simulink model "dbuildv3p2"  (R2024b)
settings: Solver=FixedStepAuto  StartTime=0.0  StopTime=inf  FixedStep=0.001  RelTol=1e-3
model workspace (MAT data in the model file):
  A_busbar = 0.0018
  A_pack = 0.711626248
  C = 400
  C_nominal = 3
  GR = 13.75
  I_max = 157.708978328
  Izz = 76.97
  M = 251.54
  P = 5
  P_DD = 1
  REGEN_GAIN = 0
  R_e = 0.197
  S = 138
  SW_TV_GAIN = 0.0250298750679
  SoC_initial = 1
  TC_CUT = 500
  T_amb = 296.15
  Tmax = 21
  W = 1.53
  W_max = 34
  a = 0.7497
  brakebias = 0.5
  busbar_CC_area = 1.8e-05
  busbar_Cp = 237
  busbar_length = 0.1
  busbar_mass = 0.016128
  busbar_resistivity = 1.68e-08
  busbar_thermalcontact_resistance = 1
  c_factor = 0.244
  cell_Cp = 1000
  cell_mass = 0.046
  deg_to_rad = 0.0174533
  g = 9.81
  h = 0.253
  h_busbar = 5
  h_pack = 5
  kappa_thresh = 0.09
  l = 1.53
  mpersec_to_kph = 3.6
  rackdisp_to_steerangle = 1.29615626969
  rad_to_deg = 57.2958
  rpm_to_radpers = 0.10472
  t = 1.2
  trigger_pressure = 4.65396
undefined symbols (not defined in the file): TC_switch, TV_switch
libraries: eeGeneralControl x2, Solver_SF x1, sl3dlib x1, simulink x1
(part 1 of 2)
settings Model: Creator=account  LastModifiedBy=kara.28

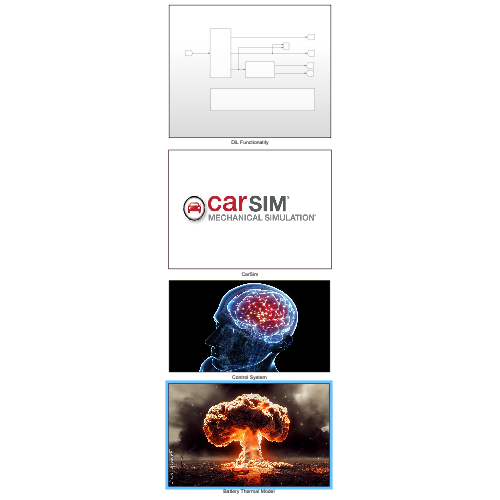
[thumbnail: Simulink's stored preview of the top-level diagram]
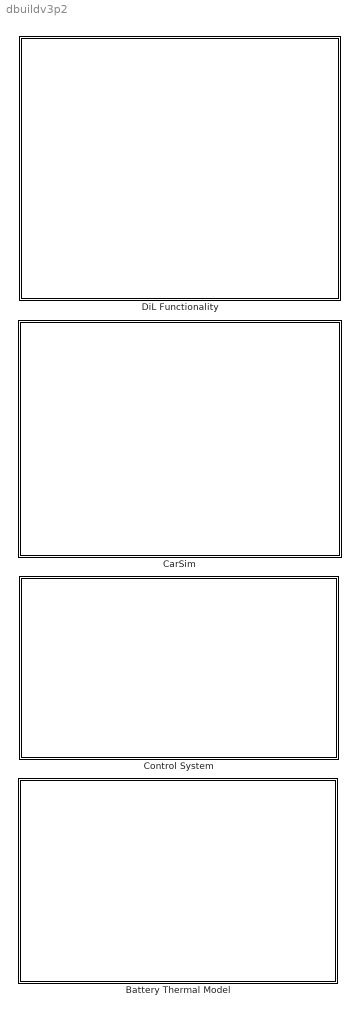
== system dbuildv3p2 ==
  Battery Thermal Model : Subsystem
      mask Display: image('battery.jpg');
  CarSim : Subsystem
      mask Display: image('carsimlogo.jpg');
  Control System : Subsystem
      mask Display: image('controller.jpg');
  DiL Functionality : Subsystem

== system dbuildv3p2/Battery Thermal Model ==
  Air Temp : Subsystem
  Battery Cells : Subsystem
  Bus Bars : Subsystem

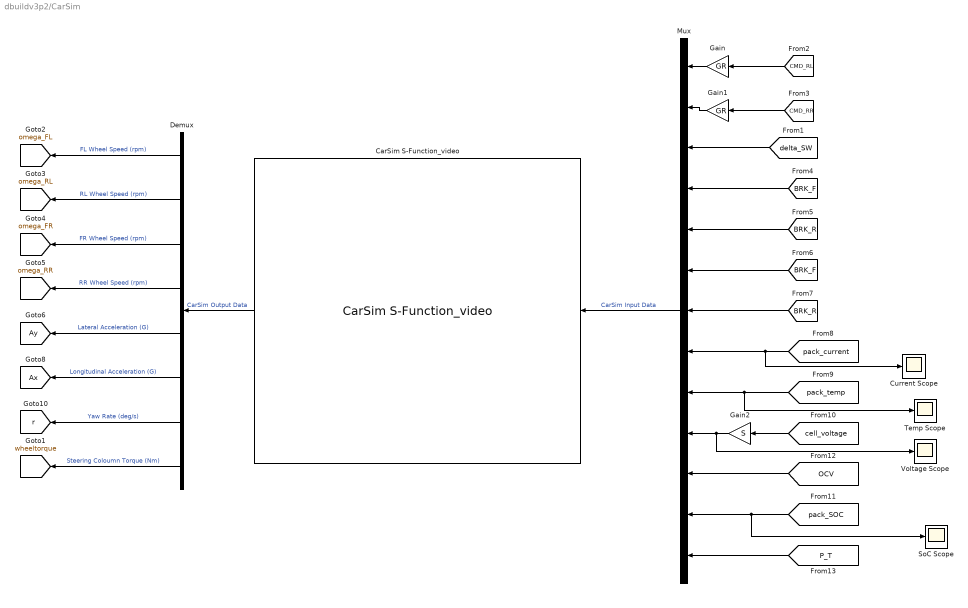
== system dbuildv3p2/CarSim ==
  CarSim S-Function_video : Solver_SF/CarSim S-Function_video  Priority=1  SIMFILE=simfile.sim
      settings: SourceProductName=CarSim S-Function
  Current Scope : Scope
  Demux : Demux  Outputs=8
  Gain : Gain  Gain=GR
  Gain1 : Gain  Gain=GR
  Gain2 : Gain  Gain=S
  Mux : Mux  Inputs=13
  SoC Scope : Scope
  Temp Scope : Scope
  Voltage Scope : Scope
  tag scope: Ax=global, Ay=global, omega_FL=global, omega_FR=global, omega_RL=global, omega_RR=global, r=global, wheeltorque=global
  wires:
  CarSim S-Function_video/1 -> Demux/1  "CarSim Output Data"
  [BRK_F] -> Mux/6
  Gain/1 -> Mux/1
  [pack_current] -> Current Scope/1, Mux/8
  Mux/1 -> CarSim S-Function_video/1  "CarSim Input Data"
  [BRK_R] -> Mux/7
  Gain1/1 -> Mux/2
  [BRK_R] -> Mux/5
  [BRK_F] -> Mux/4
  [delta_SW] -> Mux/3
  Demux/1 -> [omega_FL]  "FL Wheel Speed (rpm)"
  Demux/2 -> [omega_RL]  "RL Wheel Speed (rpm)"
  Demux/3 -> [omega_FR]  "FR Wheel Speed (rpm)"
  Demux/4 -> [omega_RR]  "RR Wheel Speed (rpm)"
  Demux/5 -> [Ay]  "Lateral Acceleration (G)"
  Demux/6 -> [Ax]  "Longitudinal Acceleration (G)"
  Demux/7 -> [r]  "Yaw Rate (deg/s)"
  Demux/8 -> [wheeltorque]  "Steering Coloumn Torque (Nm)"
  [pack_SOC] -> SoC Scope/1, Mux/12
  [OCV] -> Mux/11
  [cell_voltage] -> Gain2/1
  [pack_temp] -> Temp Scope/1, Mux/9
  Gain2/1 -> Voltage Scope/1, Mux/10
  [CMD_RL] -> Gain/1
  [CMD_RR] -> Gain1/1
  [P_T] -> Mux/13

== system dbuildv3p2/Control System ==
  Driver Assists : Subsystem
      settings: PortSchema="{\"entries\":[{\"content\":{\"sides\":[{\"content\":{\"connectorIds\":[\"In1\",\"In2\"]},\"type\":\"ConnectorPlacement.EquallySpacedRectSide\",\"uuid\":\"c30f5bbb-5f7b-4b8f-a220-579b9cc0865f\"},{\"content\":{\"connectorIds\":[\"Out1\",\"Out2\"],\"side\":\"RIGHT\"},\"type\":\"ConnectorPlacement.EquallySpacedRectSide\",\"uuid\":\"8399a92e-19c3-49c4-801c-f7e7f76799cf\"},{\"content\":{\"connectorIds\":[\"In3\",\"In4\",\"In5\",\"In6\",\"In7\",\"In8\",\"In9\"],\"side\":\"TOP\"},\"type\":\"ConnectorPlacement.EquallySpacedRectSide\",\"uuid\":\"19d8375b-8353-4f23-adee-fcd0b0fbd4ef\"}]},\"type\":\"ConnectorPlacement.EquallySpacedConnector\",\"uuid\":\"53834b5a-6686-42bc-a078-9cae71bfd001\"}],\"packageUris\":[\"http://schema.mathworks.com/mf0/Connector/R2020b\"],\"version\":\"1.0\"}"
  Dynamic Derate Dial Position : Constant  Value=3
  Energy Management System : Subsystem
      settings: PortSchema="{\"entries\":[{\"content\":{\"sides\":[{\"content\":{\"connectorIds\":[\"In1\",\"In2\"]},\"type\":\"ConnectorPlacement.EquallySpacedRectSide\",\"uuid\":\"89c92abe-ca77-4c48-ba79-1fd8447b36ee\"},{\"content\":{\"connectorIds\":[\"Out1\",\"Out2\"],\"side\":\"RIGHT\"},\"type\":\"ConnectorPlacement.EquallySpacedRectSide\",\"uuid\":\"4a58accb-bbe3-490f-b1ea-5257f75ab2ba\"},{\"content\":{\"connectorIds\":[\"In3\",\"In4\",\"In5\"],\"side\":\"TOP\"},\"type\":\"ConnectorPlacement.EquallySpacedRectSide\",\"uuid\":\"b5e96e52-1098-4ccd-9740-b2b10d8cf6b3\"}]},\"type\":\"ConnectorPlacement.EquallySpacedConnector\",\"uuid\":\"06c6d35a-fc7b-4382-b862-8bbe65743431\"}],\"packageUris\":[\"http://schema.mathworks.com/mf0/Connector/R2020b\"],\"version\":\"1.0\"}"
  tag scope: CMD_RL=global, CMD_RR=global
  wires:
  Energy Management System/1(CMD_R) -> Driver Assists/1(CMD_R)
  Energy Management System/2(Tmax) -> Driver Assists/2(Tmax)
  Driver Assists/1(CMD_RL) -> [CMD_RL]
  Driver Assists/2(CMD_RR) -> [CMD_RR]
  [pack_temp] -> Energy Management System/1(T_BAT_MAX)  "Battery Temp (C)"
  Dynamic Derate Dial Position/1 -> Energy Management System/2(P_DD)  "Derate Dial Position (-)"
  [omega_RR] -> Driver Assists/6(omega_RR), Energy Management System/5(omega_RR)  "RR Wheel Speed (rpm)"
  [omega_FR] -> Driver Assists/4(omega_FR)  "FR Wheel Speed (rpm)"
  [omega_RL] -> Driver Assists/5(omega_RL), Energy Management System/3(omega_RL)  "RL Wheel Speed (rpm)"
  [omega_FL] -> Driver Assists/3(omega_FL)  "FL Wheel Speed (rpm)"
  [P_T] -> Driver Assists/7(P_T)  "Throttle Position (-)"
  [Ay] -> Driver Assists/8(Ax)  "Lateral Acceleration (G)"
  [BRK_F] -> Driver Assists/9(BRK_F), Energy Management System/4(BRK_F)  "Front Brake Pressure (MPa)"

== system dbuildv3p2/DiL Functionality ==
  Brake system : Subsystem
  Driver inputs : Subsystem
  Real Time Sync : Subsystem
  Scope : Scope  NumInputPorts=2
  tag scope: BRK_F=global, BRK_R=global, P_T=global, delta_SW=global
  wires:
  Driver inputs/2(Throttle %) -> Scope/1, [P_T]  "Throttle (-)"
  Driver inputs/1(Steering) -> [delta_SW]  "Steering Angle (deg)"
  [wheeltorque] -> Driver inputs/1(Wheel torque)
  Brake system/1(Front brake pressure) -> [BRK_F]  "Front Brake Pressure (MPa)"
  Brake system/2(Rear brake pressure) -> [BRK_R]  "Front Brake Pressure (MPa)"
  Driver inputs/3(Brake %) -> Brake system/1(brake %), Scope/2  "Brake (-)"

== system dbuildv3p2/Battery Thermal Model/Air Temp ==
  Constant : Constant  Value=0.25
  Constant1 : Constant  Value=1005
  Constant2 : Constant  Value=T_amb
  Divide : Product  Inputs=*/
  Integrator : Integrator
  Product : Product
  Sum : Sum  Inputs=|++
  tag scope: airtemp=global
  wires:
  [pack_heatloss] -> Divide/1
  Product/1 -> Divide/2
  Constant/1 -> Product/2
  Constant1/1 -> Product/1
  Divide/1 -> Integrator/1
  Integrator/1 -> Sum/1
  Constant2/1 -> Sum/2
  Sum/1 -> [airtemp]

== system dbuildv3p2/Battery Thermal Model/Battery Cells ==
  Battery Heat : Subsystem
      settings: PortSchema="{\"entries\":[{\"content\":{\"sides\":[{\"content\":{\"connectorIds\":[\"In1\",\"Out1\",\"In2\"]},\"type\":\"ConnectorPlacement.EquallySpacedRectSide\",\"uuid\":\"0f7c0562-63f7-413a-9c65-7d5d0f23ac53\"},{\"content\":{\"side\":\"RIGHT\"},\"type\":\"ConnectorPlacement.EquallySpacedRectSide\",\"uuid\":\"6856fc4a-e601-47fb-aafe-3183d6398fa2\"},{\"content\":{\"side\":\"TOP\"},\"type\":\"ConnectorPlacement.EquallySpacedRectSide\",\"uuid\":\"93500152-ab0c-4e86-a765-8796b82b9cd6\"}]},\"type\":\"ConnectorPlacement.EquallySpacedConnector\",\"uuid\":\"8bef09a8-0835-4033-ba4e-3f5f6277d0ac\"}],\"packageUris\":[\"http://schema.mathworks.com/mf0/Connector/R2020b\"],\"version\":\"1.0\"}"
  Battery Heat Generation : Subsystem
  Heat Loss : Subsystem
      settings: PortSchema="{\"entries\":[{\"content\":{\"sides\":[{\"content\":{},\"type\":\"ConnectorPlacement.EquallySpacedRectSide\",\"uuid\":\"cd11f8f0-ebc0-4dda-8c98-00f5919de41a\"},{\"content\":{\"connectorIds\":[\"In1\",\"Out1\"],\"side\":\"RIGHT\"},\"type\":\"ConnectorPlacement.EquallySpacedRectSide\",\"uuid\":\"2a68a9a1-bd97-4a17-8a8b-1aa98e9bd9a8\"},{\"content\":{\"side\":\"TOP\"},\"type\":\"ConnectorPlacement.EquallySpacedRectSide\",\"uuid\":\"debcc510-941b-4448-a371-f67c84c59f32\"}]},\"type\":\"ConnectorPlacement.EquallySpacedConnector\",\"uuid\":\"91559e46-754b-48b4-ac3e-ab135f9add0a\"}],\"packageUris\":[\"http://schema.mathworks.com/mf0/Connector/R2020b\"],\"version\":\"1.0\"}"
  wires:
  Battery Heat/1(Pack Temp (K)) -> Heat Loss/1(Pack Temp (K))
  Battery Heat Generation/1(Battery Heat Generation Rate) -> Battery Heat/1(Battery Heat Generation)
  Heat Loss/1(Pack Heat Loss Rate) -> Battery Heat/2(Battery Heat Loss)

== system dbuildv3p2/Battery Thermal Model/Bus Bars ==
  Ambient Heat Loss : Subsystem
      settings: PortSchema="{\"entries\":[{\"content\":{\"sides\":[{\"content\":{},\"type\":\"ConnectorPlacement.EquallySpacedRectSide\",\"uuid\":\"cd11f8f0-ebc0-4dda-8c98-00f5919de41a\"},{\"content\":{\"connectorIds\":[\"In1\",\"Out1\"],\"side\":\"RIGHT\"},\"type\":\"ConnectorPlacement.EquallySpacedRectSide\",\"uuid\":\"2a68a9a1-bd97-4a17-8a8b-1aa98e9bd9a8\"},{\"content\":{\"side\":\"TOP\"},\"type\":\"ConnectorPlacement.EquallySpacedRectSide\",\"uuid\":\"debcc510-941b-4448-a371-f67c84c59f32\"}]},\"type\":\"ConnectorPlacement.EquallySpacedConnector\",\"uuid\":\"91559e46-754b-48b4-ac3e-ab135f9add0a\"}],\"packageUris\":[\"http://schema.mathworks.com/mf0/Connector/R2020b\"],\"version\":\"1.0\"}"
  Busbar Heat : Subsystem
      settings: PortSchema="{\"entries\":[{\"content\":{\"sides\":[{\"content\":{\"connectorIds\":[\"In1\",\"Out1\",\"In2\"]},\"type\":\"ConnectorPlacement.EquallySpacedRectSide\",\"uuid\":\"0f7c0562-63f7-413a-9c65-7d5d0f23ac53\"},{\"content\":{\"side\":\"RIGHT\"},\"type\":\"ConnectorPlacement.EquallySpacedRectSide\",\"uuid\":\"6856fc4a-e601-47fb-aafe-3183d6398fa2\"},{\"content\":{\"side\":\"TOP\"},\"type\":\"ConnectorPlacement.EquallySpacedRectSide\",\"uuid\":\"93500152-ab0c-4e86-a765-8796b82b9cd6\"}]},\"type\":\"ConnectorPlacement.EquallySpacedConnector\",\"uuid\":\"8bef09a8-0835-4033-ba4e-3f5f6277d0ac\"}],\"packageUris\":[\"http://schema.mathworks.com/mf0/Connector/R2020b\"],\"version\":\"1.0\"}"
  Resistance Heat Generation : Subsystem
  wires:
  Ambient Heat Loss/1(Busbar Heat Loss Rate) -> Busbar Heat/2(Busbar Heat Loss)
  Resistance Heat Generation/1(Busbar Heat Generation Rate) -> Busbar Heat/1(Busbar Heat Generation)
  Busbar Heat/1(Busbar Temp (K)) -> Ambient Heat Loss/1(Busbar Temp (K))

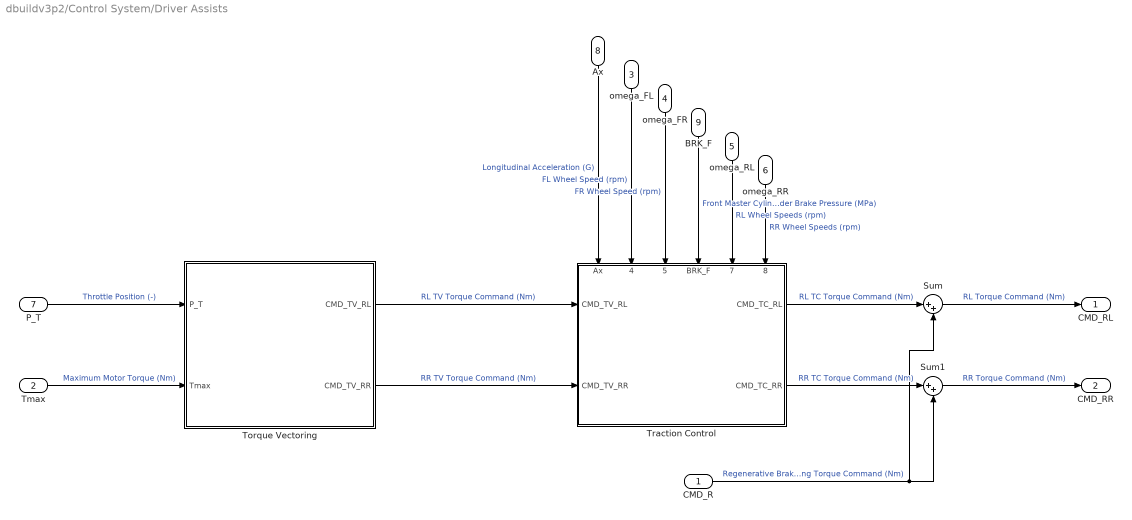
== system dbuildv3p2/Control System/Driver Assists ==
  CMD_R : Inport
  Tmax : Inport  Port=2
  omega_FL : Inport  Port=3
  omega_FR : Inport  Port=4
  omega_RL : Inport  Port=5
  omega_RR : Inport  Port=6
  P_T : Inport  Port=7
  Ax : Inport  Port=8
  BRK_F : Inport  Port=9
  Sum : Sum  Inputs=|++
  Sum1 : Sum  Inputs=|++
  Torque Vectoring : Subsystem
  Traction Control : Subsystem
      settings: PortSchema="{\"entries\":[{\"content\":{\"sides\":[{\"content\":{\"connectorIds\":[\"In1\",\"In2\"]},\"type\":\"ConnectorPlacement.EquallySpacedRectSide\",\"uuid\":\"d61c18bd-9535-4dda-869d-17effaf93de7\"},{\"content\":{\"connectorIds\":[\"Out1\",\"Out2\"],\"side\":\"RIGHT\"},\"type\":\"ConnectorPlacement.EquallySpacedRectSide\",\"uuid\":\"01ce504d-a060-4358-8411-664eedaba102\"},{\"content\":{\"connectorIds\":[\"In3\",\"In4\",\"In5\",\"In6\",\"In7\",\"In8\"],\"side\":\"TOP\"},\"type\":\"ConnectorPlacement.EquallySpacedRectSide\",\"uuid\":\"26eb6c05-86e8-47d0-a1b5-f53131bb5e60\"}]},\"type\":\"ConnectorPlacement.EquallySpacedConnector\",\"uuid\":\"a0cd41b8-03b3-4f62-a25e-73ac641935b2\"}],\"packageUris\":[\"http://schema.mathworks.com/mf0/Connector/R2020b\"],\"version\":\"1.0\"}"
  CMD_RL : Outport
  CMD_RR : Outport  Port=2
  wires:
  Torque Vectoring/2(CMD_TV_RR) -> Traction Control/2(CMD_TV_RR)  "RR TV Torque Command (Nm)"
  P_T/1 -> Torque Vectoring/1(P_T)  "Throttle Position (-)"
  Tmax/1 -> Torque Vectoring/2(Tmax)  "Maximum Motor Torque (Nm)"
  Sum/1 -> CMD_RL/1  "RL Torque Command (Nm)"
  Sum1/1 -> CMD_RR/1  "RR Torque Command (Nm)"
  CMD_R/1 -> Sum/2, Sum1/2  "Regenerative Braking Torque Command (Nm)"
  Ax/1 -> Traction Control/3(Ax)  "Longitudinal Acceleration (G)"
  omega_FL/1 -> Traction Control/4(omega_FL)  "FL Wheel Speed (rpm)"
  omega_FR/1 -> Traction Control/5(omega_FR)  "FR Wheel Speed (rpm)"
  BRK_F/1 -> Traction Control/6(BRK_F)  "Front Master Cylinder Brake Pressure (MPa)"
  omega_RL/1 -> Traction Control/7(omega_RL)  "RL Wheel Speeds (rpm)"
  omega_RR/1 -> Traction Control/8(omega_RR)  "RR Wheel Speeds (rpm)"
  Torque Vectoring/1(CMD_TV_RL) -> Traction Control/1(CMD_TV_RL)  "RL TV Torque Command (Nm)"
  Traction Control/1(CMD_TC_RL) -> Sum/1  "RL TC Torque Command (Nm)"
  Traction Control/2(CMD_TC_RR) -> Sum1/1  "RR TC Torque Command (Nm)"

== system dbuildv3p2/Control System/Energy Management System ==
  T_BAT_MAX : Inport
  P_DD : Inport  Port=2
  omega_RL : Inport  Port=3
  BRK_F : Inport  Port=4
  omega_RR : Inport  Port=5
  Dynamic Derate : Subsystem
  Regenerative Braking : Subsystem
  CMD_R : Outport
  Tmax : Outport  Port=2
  wires:
  T_BAT_MAX/1 -> Dynamic Derate/1(T_BAT_MAX)  "Maximum Module Temp (C)"
  P_DD/1 -> Dynamic Derate/2(P_DD)  "Dynamic Derate Dial Position (-)"
  BRK_F/1 -> Regenerative Braking/1(BRK_F)  "Front Master Cylinder Pressure (MPa)"
  Dynamic Derate/1(Tmax) -> Tmax/1  "Maximum Motor Torque (Nm)"
  Regenerative Braking/1(CMD_R) -> CMD_R/1  "Regen Brake Torque Command (Nm)"
  omega_RL/1 -> Dynamic Derate/3(omega_RL)  "RL Wheel Speed (rpm)"
  omega_RR/1 -> Dynamic Derate/4(omega_RR)  "RR Wheel Speed (rpm)"

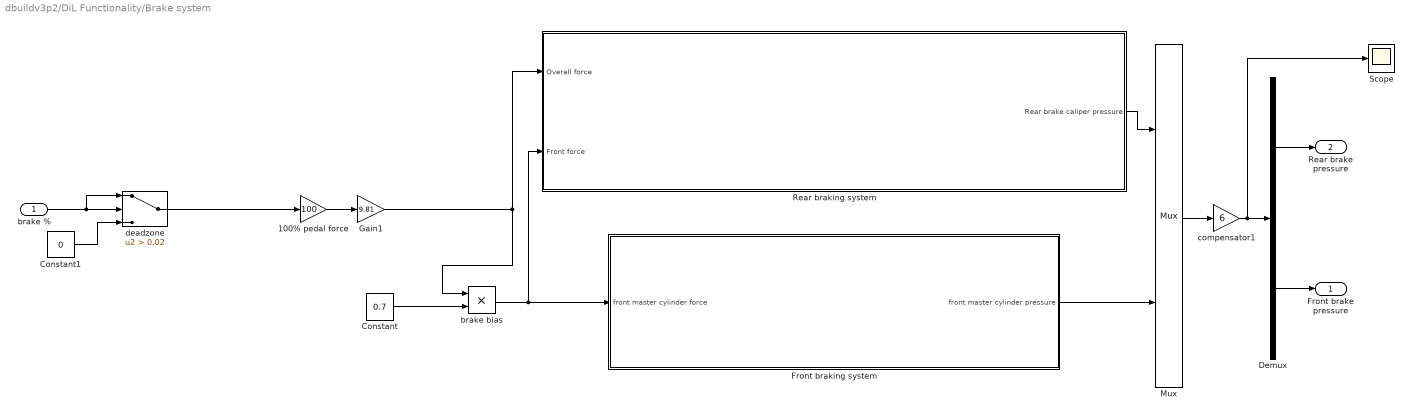
== system dbuildv3p2/DiL Functionality/Brake system ==
  brake % : Inport
  100% pedal force : Gain  Gain=100
  Constant : Constant  Value=0.7
  Constant1 : Constant  Value=0
  Demux : Demux  Outputs=2
  Front braking system : Subsystem
  Gain1 : Gain  Gain=9.81
  Mux : Mux  Inputs=2
  Rear braking system : Subsystem
  Scope : Scope
  brake bias : Product
  compensator1 : Gain  Gain=6
  deadzone : Switch  Criteria=u2 > Threshold  Threshold=0.02  SaturateOnIntegerOverflow=off  InputSameDT=off
  Front brake pressure : Outport
  Rear brake pressure : Outport  Port=2
  wires:
  100% pedal force/1 -> Gain1/1
  Constant/1 -> brake bias/2
  brake bias/1 -> Rear braking system/2(Front force), Front braking system/1(front master cylinder force)
  Gain1/1 -> brake bias/1, Rear braking system/1(Overall force)
  brake %/1 -> deadzone/1, deadzone/2
  Constant1/1 -> deadzone/3
  deadzone/1 -> 100% pedal force/1
  Rear braking system/1(Rear brake caliper pressure) -> Mux/1
  Front braking system/1(front master cylinder pressure) -> Mux/2
  Mux/1 -> compensator1/1
  compensator1/1 -> Scope/1, Demux/1
  Demux/1 -> Rear brake pressure/1
  Demux/2 -> Front brake pressure/1

== system dbuildv3p2/DiL Functionality/Driver inputs ==
  Wheel torque : Inport
  Button Box : Subsystem  Commented=on
  Simucube_Heusinkveld : Subsystem  mask{Parameter1=1, Parameter2=2, Parameter3=105}
      mask prompts: Parameter1 "Device Instance (Wheelbase)"; Parameter2 "Device Instance (Pedals)"; Parameter3 "Wheel Angle Scalar (deg)"
      mask DialogControl DescGroupVar Prompt: CarSim DS (mask) (link)
      mask DialogControl DescTextVar Prompt: Wheel and Pedal Input for CarSim/TruckSim Driving Simulator
      mask DialogControl DescTextVar Tooltip: Input 1: Force Feedback
      mask DialogControl Control2 Prompt: Input 1: Force Feedback
      mask DialogControl Control5 Prompt: Output 1: Steering Angle
      mask DialogControl Control6 Prompt: Output 2: Throttle Position (0-1)
      mask DialogControl Control7 Prompt: Output 3: Brake Position (0-1)
      mask DialogControl Control8 Prompt: Output 4: Clutch Position (0-1)
      mask DialogControl Container2 Prompt: Joystick Configuration
      mask Display: image('Simucube_Heusinkveld_Mask_1.jpg');
  Terminator : Terminator
  Steering : Outport
  Throttle % : Outport  Port=2
  Brake % : Outport  Port=3
  tag scope: TC_switch=global, TV_switch=global
  wires:
  Simucube_Heusinkveld/3(Brake) -> Brake %/1
  Simucube_Heusinkveld/4(Clutch) -> Terminator/1  "Clutch"
  Simucube_Heusinkveld/1(Steer) -> Steering/1  "Steering Angle"
  Simucube_Heusinkveld/2(Throttle) -> Throttle %/1  "throttle (-)"
  Button Box/1(TC switch) -> [TC_switch]  "TC switch"
  Button Box/2(TV switch) -> [TV_switch]  "TV switch"
  Wheel torque/1 -> Simucube_Heusinkveld/1(Force)

== system dbuildv3p2/DiL Functionality/Real Time Sync ==
  Compare To Zero : simulink/Logic and Bit Operations/Compare To Zero  relop===  OutDataTypeStr=boolean  ZeroCross=off
  Constant : Constant  Value=0
  Real-Time Synchronization Block : Subsystem  TreatAsAtomicUnit=on
  wires:
  Constant/1 -> Compare To Zero/1
  Compare To Zero/1 -> Real-Time Synchronization Block/Enable

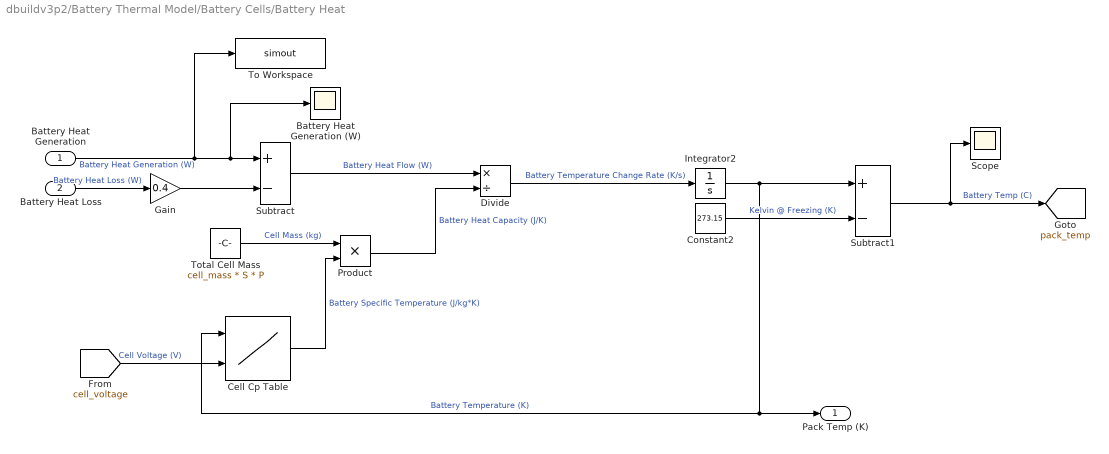
== system dbuildv3p2/Battery Thermal Model/Battery Cells/Battery Heat ==
  Battery Heat Generation : Inport
  Battery Heat Loss : Inport  Port=2
  Battery Heat Generation (W) : Scope
  Cell Cp Table : Lookup_n-D  BreakpointsForDimension1=[296.0488;303.3425;312.147;321.5769;330.6423]  BreakpointsForDimension2=[0 0.5 1]  Table=[811.0868 819.6535 830.8545;814.1373 822.704 834.6964;817.9826 826.8129 838.6737000000001;822.2249 831.0552 843.4446;826.7299 835.8239 848.3459]  InterpMethod=Cubic spline  InternalRulePriority=Speed  RndMeth=Simplest
      settings: InputPortMap=u0,u1
  Constant2 : Constant  Value=273.15
  Divide : Product  Inputs=*/
  Gain : Gain  Gain=0.4
  Integrator2 : Integrator  InitialCondition=T_amb
  Product : Product
  Scope : Scope
  Subtract : Sum  Inputs=+-
  Subtract1 : Sum  Inputs=+-
  To Workspace : ToWorkspace  VariableName=simout  SampleTime=-1
  Total Cell Mass : Constant  Value=cell_mass * S * P
  Pack Temp (K) : Outport
  tag scope: pack_temp=global
  wires:
  Cell Cp Table/1 -> Product/2  "Battery Specific Temperature (J/kg*K)"
  Constant2/1 -> Subtract1/2  "Kelvin @ Freezing (K)"
  Divide/1 -> Integrator2/1  "Battery Temperature Change Rate (K/s)"
  Subtract/1 -> Divide/1  "Battery Heat Flow (W)"
  Integrator2/1 -> Cell Cp Table/1, Pack Temp (K)/1, Subtract1/1  "Battery Temperature (K)"
  Subtract1/1 -> Scope/1, [pack_temp]  "Battery Temp (C)"
  Total Cell Mass/1 -> Product/1  "Cell Mass (kg)"
  Product/1 -> Divide/2  "Battery Heat Capacity (J/K)"
  Battery Heat Loss/1 -> Gain/1  "Battery Heat Loss (W)"
  Battery Heat Generation/1 -> To Workspace/1, Battery Heat Generation (W)/1, Subtract/1  "Battery Heat Generation (W)"
  [cell_voltage] -> Cell Cp Table/2  "Cell Voltage (V)"
  Gain/1 -> Subtract/2

== system dbuildv3p2/Battery Thermal Model/Battery Cells/Battery Heat Generation ==
  Cell Resistance : Subsystem
      settings: PortSchema="{\"entries\":[{\"content\":{\"sides\":[{\"content\":{},\"type\":\"ConnectorPlacement.EquallySpacedRectSide\",\"uuid\":\"1c6ff2a8-2c86-4b92-aa7d-5717a02d6f28\"},{\"content\":{\"connectorIds\":[\"In1\",\"In2\",\"Out1\"],\"side\":\"RIGHT\"},\"type\":\"ConnectorPlacement.EquallySpacedRectSide\",\"uuid\":\"52a4cb2c-e1db-459d-bd0a-206cc3bba6d1\"},{\"content\":{\"side\":\"TOP\"},\"type\":\"ConnectorPlacement.EquallySpacedRectSide\",\"uuid\":\"751bbbd6-abc7-4265-8d68-4aa70d69379f\"}]},\"type\":\"ConnectorPlacement.EquallySpacedConnector\",\"uuid\":\"b8f9630f-0167-4478-8d98-637e13782dcd\"}],\"packageUris\":[\"http://schema.mathworks.com/mf0/Connector/R2020b\"],\"version\":\"1.0\"}"
      mask Display: image('resistor.png');
  Cells in Parallel : Constant  Value=P
  Cells in series : Constant  Value=S
  Divide : Product  Inputs=*/
  Pack Current : Subsystem
      mask Display: image('current.png');
  Pack SoC : Subsystem
      settings: PortSchema="{\"entries\":[{\"content\":{\"sides\":[{\"content\":{},\"type\":\"ConnectorPlacement.EquallySpacedRectSide\",\"uuid\":\"1c6ff2a8-2c86-4b92-aa7d-5717a02d6f28\"},{\"content\":{\"connectorIds\":[\"In1\",\"Out1\"],\"side\":\"RIGHT\"},\"type\":\"ConnectorPlacement.EquallySpacedRectSide\",\"uuid\":\"52a4cb2c-e1db-459d-bd0a-206cc3bba6d1\"},{\"content\":{\"side\":\"TOP\"},\"type\":\"ConnectorPlacement.EquallySpacedRectSide\",\"uuid\":\"751bbbd6-abc7-4265-8d68-4aa70d69379f\"}]},\"type\":\"ConnectorPlacement.EquallySpacedConnector\",\"uuid\":\"b8f9630f-0167-4478-8d98-637e13782dcd\"}],\"packageUris\":[\"http://schema.mathworks.com/mf0/Connector/R2020b\"],\"version\":\"1.0\"}"
      mask Display: image('SoC.jpg');
  Product : Product
  Product1 : Product
  Product2 : Product
  Square : Math  Operator=square
  Battery Heat Generation Rate : Outport
  wires:
  Cells in series/1 -> Product1/1
  Divide/1 -> Cell Resistance/1(Cell Current  (A)), Square/1  "Cell Current (A)"
  Cell Resistance/1(Cell Resistance (ohms)) -> Product/2  "Cell Resistance (ohms)"
  Square/1 -> Product/1
  Cells in Parallel/1 -> Divide/2, Product1/2
  Product1/1 -> Product2/2
  Product/1 -> Product2/1  "Cell Heat Generation Rate (W)"
  Product2/1 -> Battery Heat Generation Rate/1  "Pack Heat Generation Rate (W)"
  Pack SoC/1(SoC (%)) -> Cell Resistance/2(SoC (%))  "Pack SoC (%)"
  Pack Current/1(Pack Current (A)) -> Divide/1, Pack SoC/1(Pack Current (A))  "Pack Current (A)"

== system dbuildv3p2/Battery Thermal Model/Battery Cells/Heat Loss ==
  Pack Temp (K) : Inport
  Pack Convective Heat Transfer Coefficient (W/m^2*K) : Constant  Value=h_pack
  Pack Surface Area (m^2) : Gain  Gain=A_pack
  Product : Product
  Subtract : Sum  Inputs=+-
  Pack Heat Loss Rate : Outport
  tag scope: pack_heatloss=global
  wires:
  Pack Convective Heat Transfer Coefficient (W/m^2*K)/1 -> Pack Surface Area (m^2)/1  "Pack Convective Heat Transfer Coefficient (W/m^2*K)"
  Subtract/1 -> Product/2  "Temperature Difference (K)"
  Pack Surface Area (m^2)/1 -> Product/1  "Heat Transfer Capacitance (W/K)"
  Product/1 -> [pack_heatloss], Pack Heat Loss Rate/1  "Pack Heat Loss Rate (W)"
  Pack Temp (K)/1 -> Subtract/1  "Pack Temp (K)"
  [airtemp] -> Subtract/2  "Ambient Temp (K)"

== system dbuildv3p2/Battery Thermal Model/Bus Bars/Ambient Heat Loss ==
  Busbar Temp (K) : Inport
  Air Temp Scope : Scope
  Constant : Constant  Value=273.15
  H busbar : Constant  Value=h_busbar
  Product : Product
  Subtract : Sum  Inputs=+-
  Sum : Sum  Inputs=|+-
  busbar area : Gain  Gain=A_busbar
  Busbar Heat Loss Rate : Outport
  tag scope: busbar_heatloss=global
  wires:
  [airtemp] -> Sum/1, Subtract/2
  Busbar Temp (K)/1 -> Subtract/1
  Product/1 -> Busbar Heat Loss Rate/1, [busbar_heatloss]
  busbar area/1 -> Product/1
  Subtract/1 -> Product/2
  H busbar/1 -> busbar area/1
  Sum/1 -> Air Temp Scope/1
  Constant/1 -> Sum/2

== system dbuildv3p2/Battery Thermal Model/Bus Bars/Busbar Heat ==
  Busbar Heat Generation : Inport
  Busbar Heat Loss : Inport  Port=2
  Busbar Mass : Constant  Value=busbar_mass
  Busbar Temp (C) : Scope
  Constant2 : Constant  Value=273.15
  Cp Table : Lookup_n-D  NumberOfTableDimensions=1  BreakpointsForDimension1=[300;400;600;800;1000]  Table=[401;393;379;366;352]  InterpMethod=Cubic spline  InternalRulePriority=Speed  RndMeth=Simplest
  Divide : Product  Inputs=*/
  Gain : Gain  Gain=0.1
  Gain1 : Gain
  Integrator2 : Integrator  InitialCondition=T_amb
  Product : Product
  Subtract : Sum  Inputs=+-
  Subtract1 : Sum  Inputs=+-
  Busbar Temp (K) : Outport
  tag scope: busbar_temp=global
  wires:
  Product/1 -> Gain/1
  Busbar Mass/1 -> Product/1
  Subtract1/1 -> Busbar Temp (C)/1, [busbar_temp]  "Busbar Temp (C)"
  Integrator2/1 -> Subtract1/1, Busbar Temp (K)/1, Cp Table/1
  Subtract/1 -> Divide/1
  Divide/1 -> Integrator2/1
  Constant2/1 -> Subtract1/2
  Cp Table/1 -> Product/2
  Busbar Heat Generation/1 -> Subtract/1
  Gain/1 -> Divide/2
  Busbar Heat Loss/1 -> Gain1/1
  Gain1/1 -> Subtract/2

== system dbuildv3p2/Battery Thermal Model/Bus Bars/Resistance Heat Generation ==
  Busbar cross sectional area (m^2) : Constant  Value=busbar_CC_area
  Busbar length (m) : Constant  Value=busbar_length
  Busbar resistivity (Ohms * m) : Constant  Value=busbar_resistivity
  Divide : Product  Inputs=*/
  Product : Product
  Product1 : Product
  Square : Math  Operator=square
  Busbar Heat Generation Rate : Outport
  wires:
  Divide/1 -> Product/2  "Busbar resistance (ohms)"
  Busbar cross sectional area (m^2)/1 -> Divide/2
  Product1/1 -> Divide/1
  Busbar length (m)/1 -> Product1/2
  Busbar resistivity (Ohms * m)/1 -> Product1/1
  Square/1 -> Product/1
  [pack_current] -> Square/1  "Pack Current (A)"
  Product/1 -> Busbar Heat Generation Rate/1  "Busbar Heat Gain (W)"

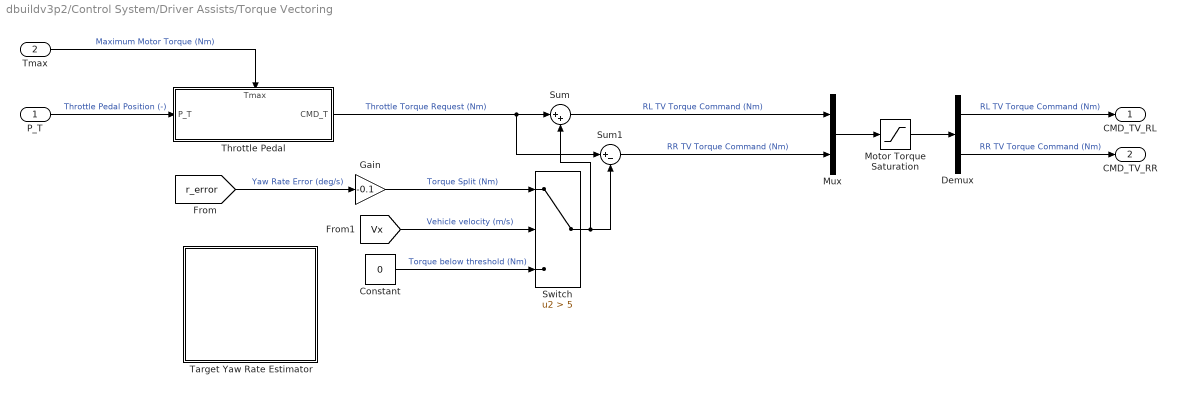
== system dbuildv3p2/Control System/Driver Assists/Torque Vectoring ==
  P_T : Inport
  Tmax : Inport  Port=2
  Constant : Constant  Value=0
  Demux : Demux  Outputs=2
  Gain : Gain  Gain=-0.1
  Motor Torque Saturation : Saturate  UpperLimit=Tmax  LowerLimit=-Tmax
  Mux : Mux  Inputs=2
  Sum : Sum  Inputs=|++
  Sum1 : Sum  Inputs=|+-
  Switch : Switch  Criteria=u2 > Threshold  Threshold=5  SaturateOnIntegerOverflow=off  InputSameDT=off
  Target Yaw Rate Estimator : Subsystem
  Throttle Pedal : Subsystem
      settings: PortSchema="{\"entries\":[{\"content\":{\"sides\":[{\"content\":{\"connectorIds\":[\"In1\"]},\"type\":\"ConnectorPlacement.EquallySpacedRectSide\",\"uuid\":\"2b27b7ae-a1b0-424c-ba89-4fa8e2fb9573\"},{\"content\":{\"connectorIds\":[\"Out1\"],\"side\":\"RIGHT\"},\"type\":\"ConnectorPlacement.EquallySpacedRectSide\",\"uuid\":\"35debb5b-e82d-4475-8dc9-1b915a5a0cae\"},{\"content\":{\"connectorIds\":[\"In2\"],\"side\":\"TOP\"},\"type\":\"ConnectorPlacement.EquallySpacedRectSide\",\"uuid\":\"f3fd2101-c365-4f42-b396-02e014a928b2\"}]},\"type\":\"ConnectorPlacement.EquallySpacedConnector\",\"uuid\":\"f19feaaa-e3f7-4392-8847-f37ac3c71c65\"}],\"packageUris\":[\"http://schema.mathworks.com/mf0/Connector/R2020b\"],\"version\":\"1.0\"}"
  CMD_TV_RL : Outport
  CMD_TV_RR : Outport  Port=2
  wires:
  Throttle Pedal/1(CMD_T) -> Sum1/1, Sum/1  "Throttle Torque Request (Nm)"
  Switch/1 -> Sum1/2, Sum/2
  Demux/1 -> CMD_TV_RL/1  "RL TV Torque Command (Nm)"
  Constant/1 -> Switch/3  "Torque below threshold (Nm)"
  Mux/1 -> Motor Torque Saturation/1
  Sum/1 -> Mux/1  "RL TV Torque Command (Nm)"
  P_T/1 -> Throttle Pedal/1(P_T)  "Throttle Pedal Position (-)"
  [r_error] -> Gain/1  "Yaw Rate Error (deg/s)"
  Motor Torque Saturation/1 -> Demux/1
  [Vx] -> Switch/2  "Vehicle velocity (m/s)"
  Tmax/1 -> Throttle Pedal/2(Tmax)  "Maximum Motor Torque (Nm)"
  Sum1/1 -> Mux/2  "RR TV Torque Command (Nm)"
  Gain/1 -> Switch/1  "Torque Split (Nm)"
  Demux/2 -> CMD_TV_RR/1  "RR TV Torque Command (Nm)"

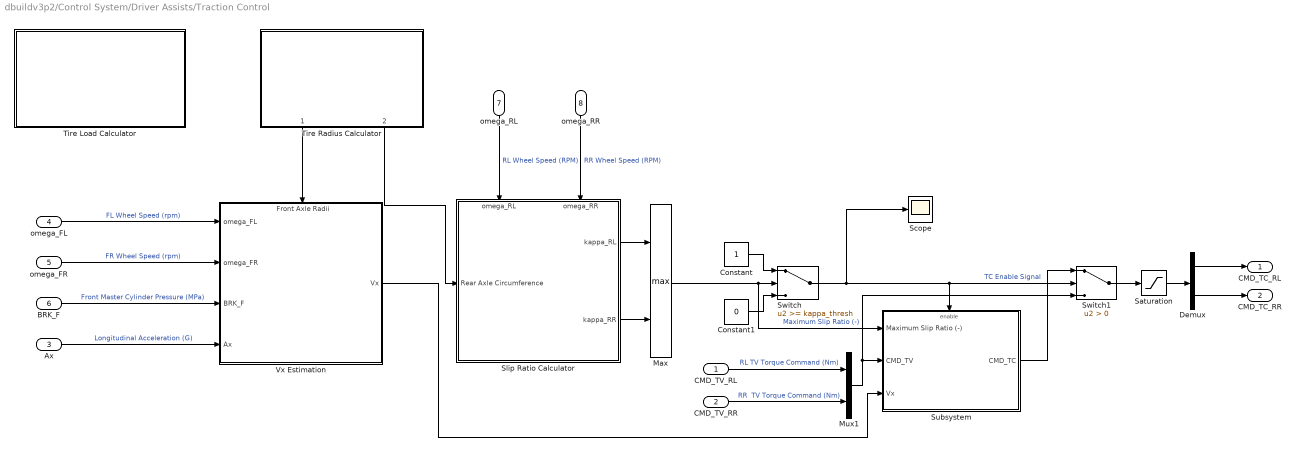
== system dbuildv3p2/Control System/Driver Assists/Traction Control ==
  CMD_TV_RL : Inport
  CMD_TV_RR : Inport  Port=2
  Ax : Inport  Port=3
  omega_FL : Inport  Port=4
  omega_FR : Inport  Port=5
  BRK_F : Inport  Port=6
  omega_RL : Inport  Port=7
  omega_RR : Inport  Port=8
  Constant : Constant
  Constant1 : Constant  Value=0
  Demux : Demux  Outputs=2
  Max : MinMax  Function=max  Inputs=2
  Mux1 : Mux  Inputs=2
  Saturation : Saturate  UpperLimit=Tmax  LowerLimit=-Tmax
  Scope : Scope
  Slip Ratio Calculator : Subsystem
      settings: PortSchema="{\"entries\":[{\"content\":{\"sides\":[{\"content\":{\"connectorIds\":[\"In1\"]},\"type\":\"ConnectorPlacement.EquallySpacedRectSide\",\"uuid\":\"7fdfdad2-33dd-4f06-b604-3c6d01a9d7f8\"},{\"content\":{\"connectorIds\":[\"Out1\",\"Out2\"],\"side\":\"RIGHT\"},\"type\":\"ConnectorPlacement.EquallySpacedRectSide\",\"uuid\":\"dd7c3b4e-ee50-4427-819e-6ce97aa41bd4\"},{\"content\":{\"connectorIds\":[\"In2\",\"In3\"],\"side\":\"TOP\"},\"type\":\"ConnectorPlacement.EquallySpacedRectSide\",\"uuid\":\"78cf20ba-e7fd-4300-9f66-06aa85c1fb42\"}]},\"type\":\"ConnectorPlacement.EquallySpacedConnector\",\"uuid\":\"f81e5908-a010-4627-83b7-5417b93ce453\"}],\"packageUris\":[\"http://schema.mathworks.com/mf0/Connector/R2020b\"],\"version\":\"1.0\"}"
  Subsystem : Subsystem
  Switch : Switch  Threshold=kappa_thresh  SaturateOnIntegerOverflow=off  InputSameDT=off
  Switch1 : Switch  Criteria=u2 > Threshold  SaturateOnIntegerOverflow=off  InputSameDT=off
  Tire Load Calculator : Subsystem
  Tire Radius Calculator : Subsystem
      settings: PortSchema="{\"entries\":[{\"content\":{\"sides\":[{\"content\":{},\"type\":\"ConnectorPlacement.EquallySpacedRectSide\",\"uuid\":\"fb3f4c67-f54c-4634-ba2d-387163a9f315\"},{\"content\":{\"side\":\"RIGHT\"},\"type\":\"ConnectorPlacement.EquallySpacedRectSide\",\"uuid\":\"aebac900-8c66-4df6-bc19-49639b103298\"},{\"content\":{\"side\":\"TOP\"},\"type\":\"ConnectorPlacement.EquallySpacedRectSide\",\"uuid\":\"62c460bb-53fa-4252-8c13-d4e682a4bd0f\"},{\"content\":{\"connectorIds\":[\"Out1\",\"Out2\"],\"side\":\"BOTTOM\"},\"type\":\"ConnectorPlacement.EquallySpacedRectSide\",\"uuid\":\"783325cb-2928-4cef-a318-c835c1a005cf\"}]},\"type\":\"ConnectorPlacement.EquallySpacedConnector\",\"uuid\":\"2844ae35-273c-4d05-aae8-a401eaebcede\"}],\"packageUris\":[\"http://schema.mathworks.com/mf0/Connector/R2020b\"],\"version\":\"1.0\"}"
  Vx Estimation : Subsystem
      settings: PortSchema="{\"entries\":[{\"content\":{\"sides\":[{\"content\":{\"connectorIds\":[\"In1\",\"In2\",\"In3\",\"In4\"]},\"type\":\"ConnectorPlacement.EquallySpacedRectSide\",\"uuid\":\"62c79b25-0b9e-432c-bd58-3f819ebc25c7\"},{\"content\":{\"connectorIds\":[\"Out1\"],\"side\":\"RIGHT\"},\"type\":\"ConnectorPlacement.EquallySpacedRectSide\",\"uuid\":\"fa527cf3-b94d-4be1-9a9d-04b034fbf641\"},{\"content\":{\"connectorIds\":[\"In5\"],\"side\":\"TOP\"},\"type\":\"ConnectorPlacement.EquallySpacedRectSide\",\"uuid\":\"a12a099b-dd90-47cf-b0e3-d9aaf4967d5c\"}]},\"type\":\"ConnectorPlacement.EquallySpacedConnector\",\"uuid\":\"1196224d-9c5e-4514-ac5e-213e9ecc2f15\"}],\"packageUris\":[\"http://schema.mathworks.com/mf0/Connector/R2020b\"],\"version\":\"1.0\"}"
  CMD_TC_RL : Outport
  CMD_TC_RR : Outport  Port=2
  wires:
  Ax/1 -> Vx Estimation/4(Ax)  "Longitudinal Acceleration (G)"
  omega_FL/1 -> Vx Estimation/1(omega_FL)  "FL Wheel Speed (rpm)"
  omega_FR/1 -> Vx Estimation/2(omega_FR)  "FR Wheel Speed (rpm)"
  BRK_F/1 -> Vx Estimation/3(BRK_F)  "Front Master Cylinder Pressure (MPa)"
  omega_RL/1 -> Slip Ratio Calculator/2(omega_RL)  "RL Wheel Speed (RPM)"
  omega_RR/1 -> Slip Ratio Calculator/3(omega_RR)  "RR Wheel Speed (RPM)"
  Vx Estimation/1(Vx) -> Subsystem/3(Vx)
  Constant/1 -> Switch/1
  Constant1/1 -> Switch/3
  Switch/1 -> Scope/1, Switch1/2, Subsystem/Enable  "TC Enable Signal"
  Subsystem/1(CMD_TC) -> Switch1/1
  CMD_TV_RL/1 -> Mux1/1  "RL TV Torque Command (Nm)"
  CMD_TV_RR/1 -> Mux1/2  "RR  TV Torque Command (Nm)"
  Mux1/1 -> Switch1/3, Subsystem/2(CMD_TV)
  Switch1/1 -> Saturation/1
  Demux/1 -> CMD_TC_RL/1
  Demux/2 -> CMD_TC_RR/1
  Max/1 -> Subsystem/1(Maximum Slip Ratio (-)), Switch/2  "Maximum Slip Ratio (-)"
  Saturation/1 -> Demux/1
  Slip Ratio Calculator/2(kappa_RR) -> Max/2
  Slip Ratio Calculator/1(kappa_RL) -> Max/1
  Tire Radius Calculator/1(Front Axle Circumference) -> Vx Estimation/5("Front Axle Radii ")
  Tire Radius Calculator/2(Rear Axle Circumference) -> Slip Ratio Calculator/1(Rear Axle Circumference)

== system dbuildv3p2/Control System/Energy Management System/Dynamic Derate ==
  T_BAT_MAX : Inport
  P_DD : Inport  Port=2
  omega_RL : Inport  Port=3
  omega_RR : Inport  Port=4
  Dynamic Derate 3D LUT : Lookup_n-D  NumberOfTableDimensions=3  BreakpointsForDimension1=[20;30;40;50;60]  BreakpointsForDimension2=[30;50;60;80]  BreakpointsForDimension3=[1 2 3 4]  Table=reshape([73.5 73.5 73.5 73.5 73.5 73.5 73.5 73.5 73.5 73.5 73.5 73.5 73.5 73.5 73.5 73.5 73.5 73.5 73.5 73.5 80 80 70 60 50 80 75 67.5 50 45 80 70 65 45 40 80 70 65 42.5 30 70 70 70 65 60 65 60 65 60 55 60 55 55 55 50 55 50 50 50 45 18.375 18.375 18.375 18.375 18.375 15 15 12.5 10 7.5 10 10 7.5 5 3.75 5 3.75 3.125 2.5 2.5], [5 4 4])  ExtrapMethod=Clip  InternalRulePriority=Speed  RndMeth=Simplest
      settings: InputPortMap=u0,u1,u2
  Gain : Gain  Gain=3.6
  Max Battery Output Limit : Scope
  Motor Output Saturation : Saturate  UpperLimit=Tmax  LowerLimit=0
  Motor Torque Calculator : Subsystem
      settings: PortSchema="{\"entries\":[{\"content\":{\"sides\":[{\"content\":{\"connectorIds\":[\"In1\",\"In2\"]},\"type\":\"ConnectorPlacement.EquallySpacedRectSide\",\"uuid\":\"904eb794-76c4-4372-ae2c-4ef2e0000433\"},{\"content\":{\"connectorIds\":[\"Out1\"],\"side\":\"RIGHT\"},\"type\":\"ConnectorPlacement.EquallySpacedRectSide\",\"uuid\":\"8161fba4-68b1-4b44-95f9-b05533d0f86a\"},{\"content\":{\"connectorIds\":[\"In3\"],\"side\":\"TOP\"},\"type\":\"ConnectorPlacement.EquallySpacedRectSide\",\"uuid\":\"e37aa600-3bd6-4b73-8bba-520f94d37a3f\"}]},\"type\":\"ConnectorPlacement.EquallySpacedConnector\",\"uuid\":\"d8616461-ce1c-4b50-a881-919f614525dd\"}],\"packageUris\":[\"http://schema.mathworks.com/mf0/Connector/R2020b\"],\"version\":\"1.0\"}"
  Scope : Scope
  Tmax : Outport
  wires:
  T_BAT_MAX/1 -> Dynamic Derate 3D LUT/1  "Maximum Module Temp (C)"
  P_DD/1 -> Dynamic Derate 3D LUT/3  "Dynamic Derate Dial Position (-)"
  Dynamic Derate 3D LUT/1 -> Max Battery Output Limit/1, Motor Torque Calculator/3(B_MAX)  "Maximum Battery Power (KW)"
  omega_RL/1 -> Motor Torque Calculator/1(omega_RL)  "RL Wheel Speed (rpm)"
  omega_RR/1 -> Motor Torque Calculator/2(omega_RR)  "RR Wheel Speed (rpm)"
  Motor Torque Calculator/1(Tmax) -> Motor Output Saturation/1  "Maximum Motor Output Torque (Nm)"
  Motor Output Saturation/1 -> Scope/1, Tmax/1
  [Vx] -> Gain/1  "Vehicle Velocity (m/s)"
  Gain/1 -> Dynamic Derate 3D LUT/2  "Vehicle Velocity (kph)"

== system dbuildv3p2/Control System/Energy Management System/Regenerative Braking ==
  BRK_F : Inport
  Regen Brake Torque Gain : Gain  Gain=-1
  CMD_R : Outport
  wires:
  BRK_F/1 -> Regen Brake Torque Gain/1  "Front Master Cylinder Pressure (MPa)"
  Regen Brake Torque Gain/1 -> CMD_R/1  "Regen Brake Torque Command (Nm)"

== system dbuildv3p2/DiL Functionality/Brake system/Front braking system ==
  front master cylinder force : Inport
  Divide : Product  Inputs=*/
  Front bore size : Constant  Value=0.625
  Gain : Gain  Gain=0.5 * pi
  Gain2 : Gain  Gain=0.00064516
  Gain3 : Gain  Gain=1e-6
  Square : Math  Operator=square
  front master cylinder pressure : Outport
  wires:
  Front bore size/1 -> Square/1
  Gain/1 -> Gain2/1
  front master cylinder force/1 -> Divide/1
  Gain2/1 -> Divide/2
  Square/1 -> Gain/1
  Divide/1 -> Gain3/1
  Gain3/1 -> front master cylinder pressure/1

== system dbuildv3p2/DiL Functionality/Brake system/Rear braking system ==
  Overall force : Inport
  Front force : Inport  Port=2
  Divide1 : Product  Inputs=*/
  Gain : Gain  Gain=0.5
  Gain4 : Gain  Gain=pi
  Gain5 : Gain  Gain=0.00064516
  Proportioning valve : Subsystem
  Rear bore size : Constant  Value=0.875
  Square1 : Math  Operator=square
  Subtract : Sum  Inputs=+-
  to mPa : Gain  Gain=1e-6
  Rear brake caliper pressure : Outport
  wires:
  Front force/1 -> Subtract/2
  Subtract/1 -> Divide1/1
  Square1/1 -> Gain4/1
  Rear bore size/1 -> Gain/1
  Gain4/1 -> Gain5/1
  Gain5/1 -> Divide1/2
  Overall force/1 -> Subtract/1
  Divide1/1 -> to mPa/1
  to mPa/1 -> Proportioning valve/1(rear master cylinder pressure)
  Proportioning valve/1(proportioning valve pressure) -> Rear brake caliper pressure/1
  Gain/1 -> Square1/1

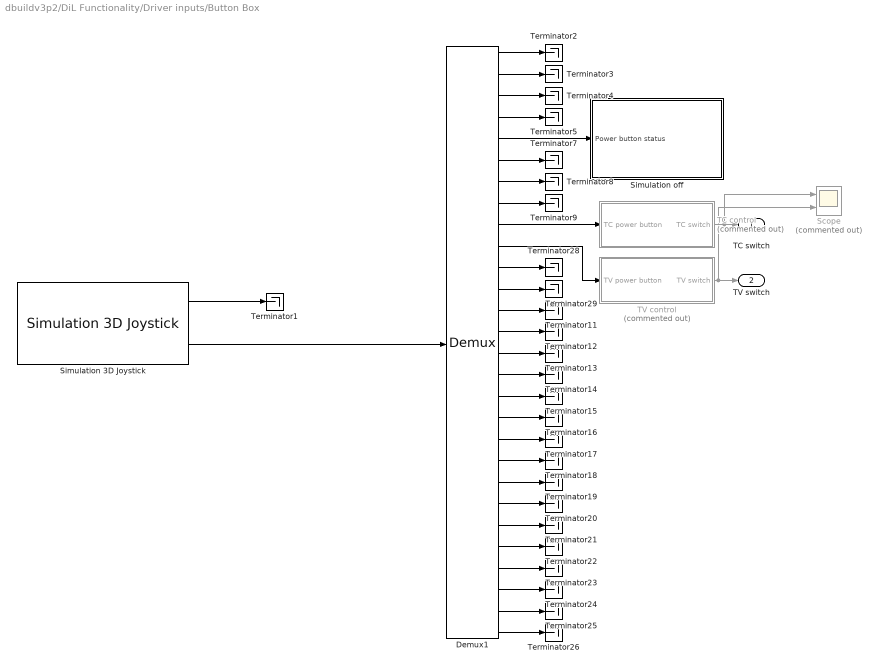
== system dbuildv3p2/DiL Functionality/Driver inputs/Button Box ==
  Demux1 : Demux  Outputs=28
  Scope : Scope  Commented=on  NumInputPorts=2
  Simulation 3D Joystick : sl3dlib/Simulation 3D/Hardware Interface/Simulation 3D Joystick  joyid=0  adjustports=off  forcefeed=off
  Simulation off : Subsystem
  TC control : Subsystem  Commented=on
  TV control : Subsystem  Commented=on
  Terminator{1..5,7..9,11..26,28..29} (26 alike) : Terminator
  TC switch : Outport
  TV switch : Outport  Port=2
  wires:
  Demux1/3 -> Terminator4/1
  Demux1/2 -> Terminator3/1
  Demux1/17 -> Terminator15/1
  Demux1/26 -> Terminator24/1
  Demux1/14 -> Terminator12/1
  Demux1/15 -> Terminator13/1
  Demux1/24 -> Terminator22/1
  Demux1/10 -> TV control/1(TV power button)
  Demux1/7 -> Terminator8/1
  Demux1/27 -> Terminator25/1
  Demux1/28 -> Terminator26/1
  Demux1/6 -> Terminator7/1
  Demux1/1 -> Terminator2/1
  Demux1/16 -> Terminator14/1
  Demux1/21 -> Terminator19/1
  Demux1/20 -> Terminator18/1
  Demux1/8 -> Terminator9/1
  Demux1/23 -> Terminator21/1
  Demux1/13 -> Terminator11/1
  Demux1/4 -> Terminator5/1
  Demux1/25 -> Terminator23/1
  Demux1/19 -> Terminator17/1
  Demux1/18 -> Terminator16/1
  Demux1/5 -> Simulation off/1(Power button status)
  Simulation 3D Joystick/1 -> Terminator1/1
  Simulation 3D Joystick/2 -> Demux1/1
  Demux1/22 -> Terminator20/1
  Demux1/12 -> Terminator29/1
  Demux1/11 -> Terminator28/1
  Demux1/9 -> TC control/1(TC power button)
  TC control/1(TC switch) -> Scope/1, TC switch/1
  TV control/1(TV switch) -> TV switch/1, Scope/2

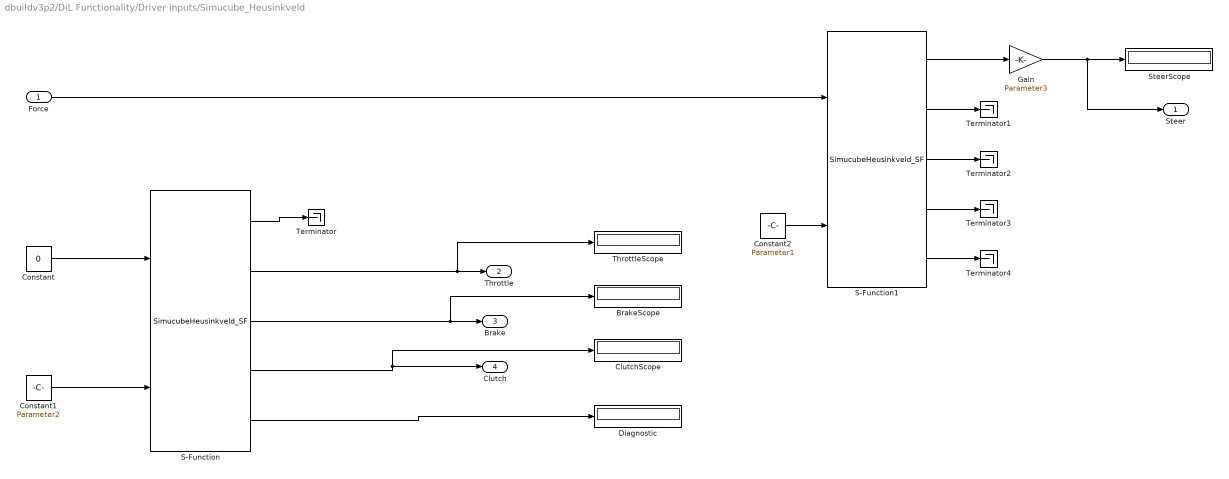
== system dbuildv3p2/DiL Functionality/Driver inputs/Simucube_Heusinkveld ==
  Force : Inport
  BrakeScope : Display
  ClutchScope : Display
  Constant : Constant  Value=0
  Constant1 : Constant  Value=Parameter2
  Constant2 : Constant  Value=Parameter1
  Diagnostic : Display
  Gain : Gain  Gain=Parameter3
  S-Function : S-Function  FunctionName=SimucubeHeusinkveld_SF  Parameters=5  SFunctionDeploymentMode=off  EnableBusSupport=off
  S-Function1 : S-Function  FunctionName=SimucubeHeusinkveld_SF  Parameters=5  SFunctionDeploymentMode=off  EnableBusSupport=off
  SteerScope : Display
  Terminator{,1..4} (5 alike) : Terminator
  ThrottleScope : Display
  Steer : Outport
  Throttle : Outport  Port=2
  Brake : Outport  Port=3
  Clutch : Outport  Port=4
  wires:
  S-Function/5 -> Diagnostic/1
  S-Function/4 -> ClutchScope/1, Clutch/1
  Force/1 -> S-Function1/1
  Constant1/1 -> S-Function/2
  Constant2/1 -> S-Function1/2
  S-Function1/1 -> Gain/1
  Gain/1 -> Steer/1, SteerScope/1
  S-Function/1 -> Terminator/1
  S-Function1/2 -> Terminator1/1
  S-Function1/3 -> Terminator2/1
  S-Function1/4 -> Terminator3/1
  S-Function1/5 -> Terminator4/1
  Constant/1 -> S-Function/1
  S-Function/2 -> ThrottleScope/1, Throttle/1
  S-Function/3 -> BrakeScope/1, Brake/1

== system dbuildv3p2/DiL Functionality/Real Time Sync/Real-Time Synchronization Block ==
  Enable : EnablePort
  Terminator : Terminator
  Timer for Real-Time : S-Function  FunctionName=sfun_rttime  Parameters=1  SFunctionDeploymentMode=off  EnableBusSupport=off
  wires:
  Timer for Real-Time/1 -> Terminator/1

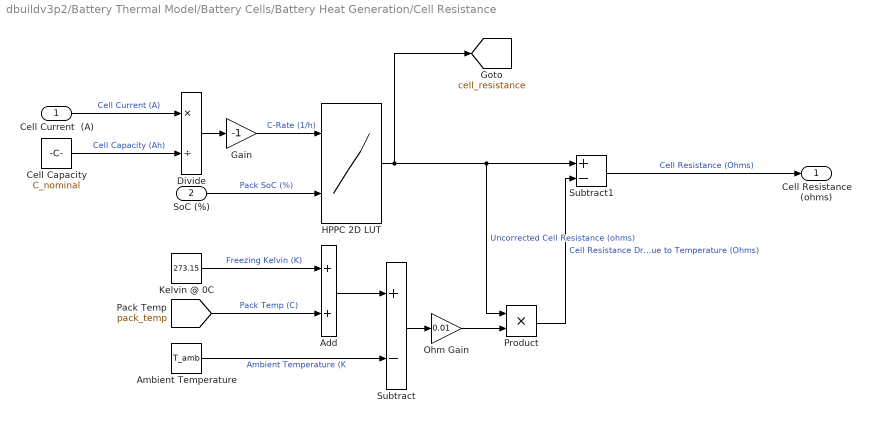
== system dbuildv3p2/Battery Thermal Model/Battery Cells/Battery Heat Generation/Cell Resistance ==
  Cell Current  (A) : Inport
  SoC (%) : Inport  Port=2
  Add : Sum
  Ambient Temperature : Constant  Value=T_amb
  Cell Capacity : Constant  Value=C_nominal
  Divide : Product  Inputs=*/
  Gain : Gain  Gain=-1
  HPPC 2D LUT : Lookup_n-D  BreakpointsForDimension1=[-10;-5;-1;1;2;3]  BreakpointsForDimension2=[0.1;0.2;0.3;0.4;0.5;0.6;0.7;0.8;0.9;1]  Table=[0.018906 0.01868 0.018453 0.018226 0.017999 0.017916 0.017743 0.018183 0.019549 0.022703;0.021356 0.020344 0.019332 0.019017 0.018694 0.018598 0.018319 0.018773 0.020642 0.024917;0.02305 0.020909 0.018859 0.019644 0.019687 0.018989 0.018291 0.019295 0.021608 0.026536;0.023001 0.020599 0.019683 0.019161 0.01894 0.018506 0.018636 0.019336 0.020993 0.02265;0.022654 0.020712 0.018901 0.018682 0.018442 0.018289 0.017788 0.017286 0.016785 0.016283;0.019898 0.017891 0.017366 0.01725 0.01725 0.017251 0.017251 0.017251 0.017251 0.017251]  InterpMethod=Cubic spline  ExtrapMethod=Clip  InternalRulePriority=Speed  RndMeth=Simplest
      settings: InputPortMap=u0,u1
  Kelvin @ 0C : Constant  Value=273.15
  Ohm Gain : Gain  Gain=0.01
  Product : Product
  Subtract : Sum  Inputs=+-
  Subtract1 : Sum  Inputs=+-
  Cell Resistance (ohms) : Outport
  tag scope: cell_resistance=global
  wires:
  Cell Current  (A)/1 -> Divide/1  "Cell Current (A)"
  Cell Capacity/1 -> Divide/2  "Cell Capacity (Ah)"
  SoC (%)/1 -> HPPC 2D LUT/2  "Pack SoC (%)"
  HPPC 2D LUT/1 -> [cell_resistance], Subtract1/1, Product/1  "Uncorrected Cell Resistance (ohms)"
  Divide/1 -> Gain/1
  Gain/1 -> HPPC 2D LUT/1  "C-Rate (1/h)"
  Subtract/1 -> Ohm Gain/1
  Ambient Temperature/1 -> Subtract/2  "Ambient Temperature (K"
  [pack_temp] -> Add/2  "Pack Temp (C)"
  Add/1 -> Subtract/1
  Kelvin @ 0C/1 -> Add/1  "Freezing Kelvin (K)"
  Ohm Gain/1 -> Product/2
  Product/1 -> Subtract1/2  "Cell Resistance Drop Due to Temperature (Ohms)"
  Subtract1/1 -> Cell Resistance (ohms)/1  "Cell Resistance (Ohms)"

== system dbuildv3p2/Battery Thermal Model/Battery Cells/Battery Heat Generation/Pack Current ==
  Divide : Product  Inputs=*/
  Gain : Gain  Gain=S
  Power Estimator : Subsystem
  Sony VTC6 Equivalent Circuit : Subsystem
  To File : ToFile  Filename=pack_current.mat  SampleTime=0.01
  Pack Current (A) : Outport
  tag scope: pack_current=global
  wires:
  Power Estimator/1(Motor Power (W)) -> Divide/1  "Driver Power Request (W)"
  Gain/1 -> Divide/2  "Pack Voltage (V)"
  Sony VTC6 Equivalent Circuit/1(Cell Voltage (V)) -> Gain/1  "Cell Voltage (V)"
  Divide/1 -> To File/1, [pack_current], Pack Current (A)/1  "Pack Current (A)"

== system dbuildv3p2/Battery Thermal Model/Battery Cells/Battery Heat Generation/Pack SoC ==
  Pack Current (A) : Inport
  Constant : Constant  Value=SoC_initial
  Constant1 : Constant  Value=P
  Divide : Product  Inputs=*/
  Gain : Gain  Gain=1/3600
  Integrator : Integrator
  Multiply : Gain  Gain=C_nominal
  Subtract : Sum  Inputs=+-
  SoC (%) : Outport
  tag scope: pack_SOC=global
  wires:
  Pack Current (A)/1 -> Integrator/1
  Constant/1 -> Subtract/1
  Integrator/1 -> Divide/1
  Subtract/1 -> [pack_SOC], SoC (%)/1
  Constant1/1 -> Multiply/1
  Multiply/1 -> Divide/2
  Divide/1 -> Gain/1
  Gain/1 -> Subtract/2

== system dbuildv3p2/Control System/Driver Assists/Torque Vectoring/Target Yaw Rate Estimator ==
  Gain : Gain  Gain=C*2
  Gain1 : Gain  Gain=C*2
  Gain2 : Gain  Gain=a
  Gain3 : Gain  Gain=l-a
  Gain4 : Gain  Gain=-1/Izz
  Slip Angle Estimator : Subsystem
  Sum : Sum  Inputs=|+-
  Yaw Rate Error : Subsystem
      settings: PortSchema="{\"entries\":[{\"content\":{\"sides\":[{\"content\":{},\"type\":\"ConnectorPlacement.EquallySpacedRectSide\",\"uuid\":\"b231141e-075c-44c2-9b61-2a7f1987e8f9\"},{\"content\":{\"side\":\"RIGHT\"},\"type\":\"ConnectorPlacement.EquallySpacedRectSide\",\"uuid\":\"a3423ff2-a1bd-4263-8320-fe535760aa80\"},{\"content\":{\"connectorIds\":[\"In1\"],\"side\":\"TOP\"},\"type\":\"ConnectorPlacement.EquallySpacedRectSide\",\"uuid\":\"1adafbb7-f7c4-42e4-8eab-5e40445049e0\"}]},\"type\":\"ConnectorPlacement.EquallySpacedConnector\",\"uuid\":\"61c95f4c-4142-4f56-9fe1-ea528e3e26a5\"}],\"packageUris\":[\"http://schema.mathworks.com/mf0/Connector/R2020b\"],\"version\":\"1.0\"}"
  tag scope: r_est=global
  wires:
  Gain1/1 -> Gain3/1  "Rear Wheel Lateral Force (N)"
  [alpha_F] -> Gain/1  "Front Wheel Slip Angle (deg)"
  Gain4/1 -> [r_est], Yaw Rate Error/1(r_est)  "Target Yaw Rate (deg/s)"
  Sum/1 -> Gain4/1  "Vehicle Yaw Moment (Nm)"
  Gain2/1 -> Sum/1  "Front Yaw Moment (Nm)"
  Gain/1 -> Gain2/1  "Front Wheel Lateral Force (N)"
  Gain3/1 -> Sum/2  "Rear Yaw Moment (Nm)"
  [alpha_R] -> Gain1/1  "Rear Wheel Slip Angle (deg)"

== system dbuildv3p2/Control System/Driver Assists/Torque Vectoring/Throttle Pedal ==
  P_T : Inport
  Tmax : Inport  Port=2
  Product : Product
  CMD_T : Outport
  wires:
  P_T/1 -> Product/2  "Throttle Pedal Position (-)"
  Product/1 -> CMD_T/1  "Throttle Pedal Torque Command (Nm)"
  Tmax/1 -> Product/1  "Maximum Motor Torque (Nm)"

== system dbuildv3p2/Control System/Driver Assists/Traction Control/Slip Ratio Calculator ==
  Rear Axle Circumference : Inport
  omega_RL : Inport  Port=2
  omega_RR : Inport  Port=3
  Abs : Abs  SaturateOnIntegerOverflow=off
  Demux : Demux  Outputs=2
  Divide : Product  Inputs=*/
  Gain : Gain  Gain=1/60
  Minus : Sum  Inputs=+-
  Mux : Mux  Inputs=2
  Product : Product
  Wheel Center Speed Calculator : Subsystem
  kappa_RL : Outport
  kappa_RR : Outport  Port=2
  wires:
  omega_RL/1 -> Mux/1
  omega_RR/1 -> Mux/2
  Mux/1 -> Gain/1  "Tire Rotational Speed (rpm)"
  Gain/1 -> Product/1  "Tire Rotational Speed (rps)"
  Demux/1 -> kappa_RL/1  "Calculated RL Slip Ratio (-)"
  Demux/2 -> kappa_RR/1  "Calculated RR Slip Ratio (-)"
  Product/1 -> Minus/1  "Tire Velocity (m/s)"
  Minus/1 -> Divide/1  "Calculated Slip Ratio (-)"
  Divide/1 -> Demux/1
  Abs/1 -> Divide/2
  Wheel Center Speed Calculator/1(Calculated Wheel Center Velocity (m/s)) -> Minus/2, Abs/1  "Calculated Wheel Center Velocity"
  Rear Axle Circumference/1 -> Product/2

== system dbuildv3p2/Control System/Driver Assists/Traction Control/Subsystem ==
  Maximum Slip Ratio (-) : Inport
  CMD_TV : Inport  Port=2
  Vx : Inport  Port=3
  Enable : EnablePort
  Constant : Constant  Value=kappa_thresh
  Constant1 : Constant  Value=0
  Gain : Gain  Gain=TC_CUT
  Saturation : Saturate  UpperLimit=0  LowerLimit=-Tmax
  Saturation1 : Saturate  UpperLimit=Tmax  LowerLimit=0
  Sum : Sum  Inputs=|+-
  Sum1 : Sum  Inputs=|++
  Sum2 : Sum  Inputs=|+-
  Switch : Switch  Criteria=u2 > Threshold  SaturateOnIntegerOverflow=off  InputSameDT=off
  Switch1 : Switch  Criteria=u2 > Threshold  SaturateOnIntegerOverflow=off  InputSameDT=off
  CMD_TC : Outport
  wires:
  Switch/1 -> CMD_TC/1  "TC Torque Command (Nm)"
  Maximum Slip Ratio (-)/1 -> Sum/1  "Maximum Slip Ratio (-)"
  Constant/1 -> Sum/2  "Target Slip Ratio (-)"
  Sum/1 -> Gain/1  "Slip Error (-)"
  CMD_TV/1 -> Sum2/1, Switch/2, Sum1/1  "TV Torque Command (Nm)"
  Vx/1 -> Switch1/2  "Vehicle Velocity (m/s)"
  Gain/1 -> Switch1/1  "Torque Cut (Nm)"
  Constant1/1 -> Switch1/3
  Switch1/1 -> Sum2/2, Sum1/2
  Sum1/1 -> Saturation/1
  Sum2/1 -> Saturation1/1
  Saturation/1 -> Switch/3
  Saturation1/1 -> Switch/1

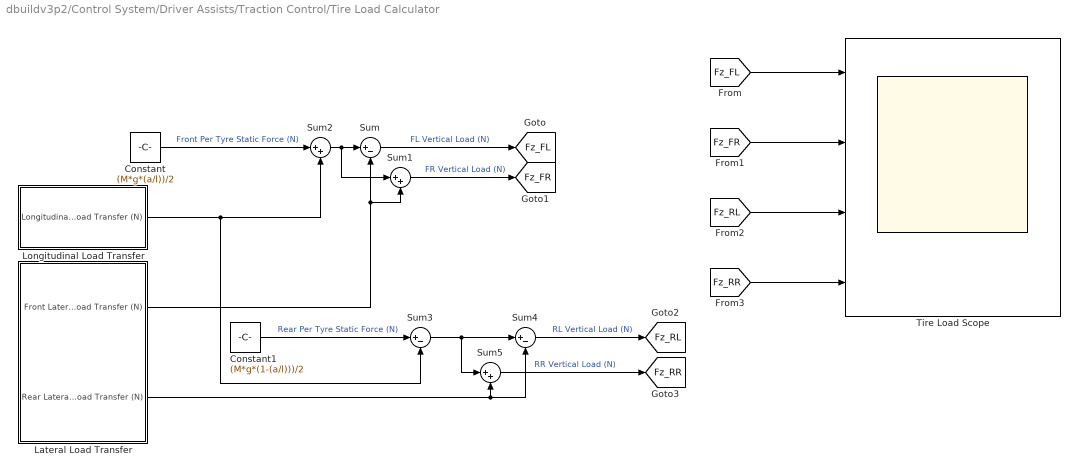
== system dbuildv3p2/Control System/Driver Assists/Traction Control/Tire Load Calculator ==
  Constant : Constant  Value=(M*g*(a/l))/2
  Constant1 : Constant  Value=(M*g*(1-(a/l)))/2
  Lateral Load Transfer : Subsystem
  Longitudinal Load Transfer : Subsystem
  Sum : Sum  Inputs=|+-
  Sum1 : Sum  Inputs=|++
  Sum2 : Sum  Inputs=|++
  Sum3 : Sum  Inputs=|+-
  Sum4 : Sum  Inputs=|+-
  Sum5 : Sum  Inputs=|++
  Tire Load Scope : Scope  NumInputPorts=4
  tag scope: Fz_FL=global, Fz_FR=global, Fz_RL=global, Fz_RR=global
  wires:
  Longitudinal Load Transfer/1(Longitudinal Load Transfer (N)) -> Sum2/2, Sum3/2
  Constant/1 -> Sum2/1  "Front Per Tyre Static Force (N)"
  Sum2/1 -> Sum1/1, Sum/1
  Lateral Load Transfer/1(Front Lateral Load Transfer (N)) -> Sum1/2, Sum/2
  Sum/1 -> [Fz_FL]  "FL Vertical Load (N)"
  Sum1/1 -> [Fz_FR]  "FR Vertical Load (N)"
  Constant1/1 -> Sum3/1  "Rear Per Tyre Static Force (N)"
  Sum3/1 -> Sum5/1, Sum4/1
  Lateral Load Transfer/2(Rear Lateral Load Transfer (N)) -> Sum4/2, Sum5/2
  Sum4/1 -> [Fz_RL]  "RL Vertical Load (N)"
  Sum5/1 -> [Fz_RR]  "RR Vertical Load (N)"
  [Fz_FL] -> Tire Load Scope/1
  [Fz_FR] -> Tire Load Scope/2
  [Fz_RL] -> Tire Load Scope/3
  [Fz_RR] -> Tire Load Scope/4

== system dbuildv3p2/Control System/Driver Assists/Traction Control/Tire Radius Calculator ==
  Constant : Constant  Value=201.094*10^-3
  Constant1 : Constant  Value=2*pi
  Demux : Demux
  Mux : Mux
  Mux1 : Mux  Inputs=2
  Mux2 : Mux  Inputs=2
  Product1 : Product
  Sum : Sum  Inputs=|++
  Tire Stiffness : Gain  Gain=-0.005509*10^-3
  Front Axle Circumference : Outport
  Rear Axle Circumference : Outport  Port=2
  wires:
  Constant1/1 -> Product1/1
  Tire Stiffness/1 -> Sum/1
  Sum/1 -> Product1/2
  Constant/1 -> Sum/2  "Unloaded Tire Radius (m)"
  Mux/1 -> Tire Stiffness/1
  [Fz_FL] -> Mux/1
  [Fz_FR] -> Mux/2
  Product1/1 -> Demux/1  "Tire Circumference (m)"
  [Fz_RL] -> Mux/3
  [Fz_RR] -> Mux/4
  Demux/1 -> Mux1/1
  Demux/4 -> Mux2/2
  Demux/3 -> Mux2/1
  Demux/2 -> Mux1/2
  Mux1/1 -> Front Axle Circumference/1
  Mux2/1 -> Rear Axle Circumference/1

== system dbuildv3p2/Control System/Driver Assists/Traction Control/Vx Estimation ==
  omega_FL : Inport
  omega_FR : Inport  Port=2
  BRK_F : Inport  Port=3
  Ax : Inport  Port=4
  "Front Axle Radii " : Inport  Port=5
  Add : Sum
  Ax to Vx : Subsystem
  Demux : Demux  Outputs=2
  Gain : Gain  Gain=0.5
  Method Enabler : Subsystem
  Mux : Mux  Inputs=2
  Velocity Method Switch : Switch  Criteria=u2 > Threshold  Threshold=0.1  SaturateOnIntegerOverflow=off  InputSameDT=off
  omega to Vx : Subsystem
  Vx : Outport
  tag scope: Vx=global
  wires:
  Mux/1 -> omega to Vx/1(omega)
  omega to Vx/1(Vx) -> Demux/1
  Demux/2 -> Add/2
  omega_FR/1 -> Mux/2
  omega_FL/1 -> Mux/1
  Demux/1 -> Add/1
  BRK_F/1 -> Velocity Method Switch/2, Method Enabler/1(BRK_F)
  Add/1 -> Gain/1
  Gain/1 -> Velocity Method Switch/3, Ax to Vx/2(Omega Vx)  "omega Vx"
  Velocity Method Switch/1 -> [Vx], Vx/1  "Vx estimated"
  Ax/1 -> Ax to Vx/1(Ax)
  Ax to Vx/1(Ax Vx) -> Velocity Method Switch/1  "Ax Vx"
  Method Enabler/2(Enable omega method) -> omega to Vx/Enable
  Method Enabler/1(Enable Ax method) -> Ax to Vx/Enable
  "Front Axle Radii "/1 -> omega to Vx/2(Front Axle Circumference)

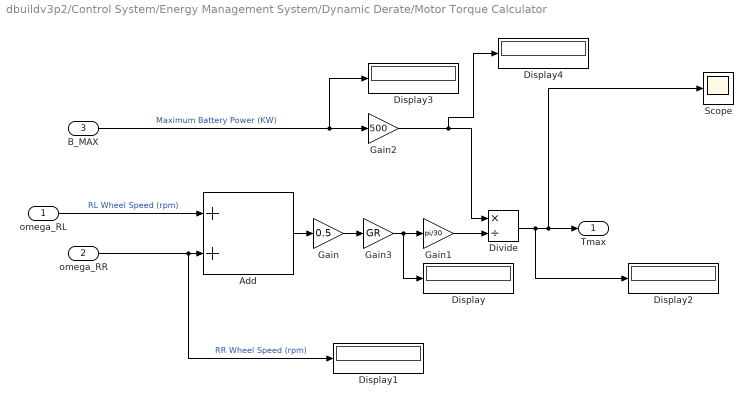
== system dbuildv3p2/Control System/Energy Management System/Dynamic Derate/Motor Torque Calculator ==
  omega_RL : Inport
  omega_RR : Inport  Port=2
  B_MAX : Inport  Port=3
  Add : Sum
  Display{,1..4} (5 alike) : Display
  Divide : Product  Inputs=*/
  Gain : Gain  Gain=0.5
  Gain1 : Gain  Gain=pi/30
  Gain2 : Gain  Gain=500
  Gain3 : Gain  Gain=GR
  Scope : Scope
  Tmax : Outport
  wires:
  omega_RR/1 -> Display1/1, Add/2  "RR Wheel Speed (rpm)"
  Add/1 -> Gain/1
  omega_RL/1 -> Add/1  "RL Wheel Speed (rpm)"
  Gain/1 -> Gain3/1
  Gain1/1 -> Divide/2
  B_MAX/1 -> Display3/1, Gain2/1  "Maximum Battery Power (KW)"
  Divide/1 -> Display2/1, Scope/1, Tmax/1
  Gain2/1 -> Display4/1, Divide/1
  Gain3/1 -> Display/1, Gain1/1
